simulink model "EDLSim_proj"  (R2022b)
settings: Solver=ode23s  StartTime=0.0  StopTime=tSim  FixedStep=0.01  MaxStep=1e3  RelTol=1e-3  EnableMultiTasking=on
values from neighbouring files (symbols this model uses):
  A = [0 0 v0 ... (first row only)    [main.m]
  Aref = A-B*K    [main.m]
  B = [0;0;1]    [main.m]
  Bref = [0;0;1]    [main.m]
  D = 0.5*rho*Cd*S*v^2    [command.m]    (also in command3.m)
  e0 = 350    [main.m]
  Gama = 1    [main.m]
  Gamar = 1    [main.m]
  Gamat = 1*eye(3)    [main.m]
  Gamax = 1*eye(3)    [main.m]
  gamma0 = deg2rad(-6.6198381)    [main.m]    (also in scaling.m = gamma0/angbar)
  meanDist = 50000    [main.m]
  P = lyap(Aref',Qref)    [main.m]
  phi0 = deg2rad(23.51457)    [main.m]
  psi0 = deg2rad(18.0683)    [main.m]
  r0 = r0*1000    (= 6498270)    [main.m]    (also in scaling.m = 1.0188351238)
  r_des = 10 * 1000    (= 10000)    [main.m]
  r_e = r_e*1000    (= 6378137)    [command.m]    (also in command3.m; main.m; scaling.m = 6378.137)
  Theta = [0 0 1]    [main.m]
  theta0 = deg2rad(174.24384)    [main.m]
  Ts = 0.01    [main.m]
  tSim = T(end)    [main.m]
  v0 = v0*1000    (= 11067.15)    [main.m]    (also in scaling.m = 1)
  varDist = 5000    [main.m]
  x0 = [r0;v0;gamma0]    [main.m]    (also in scaling.m)
settings Model: Creator=Tri  LastModifiedBy=la561195
settings SolverCC: AlgebraicLoopSolver=TrustRegion
settings DataIOCC: LimitDataPoints=on  SaveFormat=Array  ReturnWorkspaceOutputs=off
settings OptimizationCC: LifeSpan=inf
settings DebuggingCC: UnconnectedInputMsg=warning  UnconnectedOutputMsg=warning  UnconnectedLineMsg=warning  SFUnexpectedBacktrackingDiag=warning  SFNoUnconditionalDefaultTransitionDiag=warning  SFExecutionAtInitializationDiag=none  SFMachineParentedDataDiag=warning  ArithmeticOperatorsInVariantConditions=warning
settings HardwareCC: ProdBitPerPointer=32  ProdBitPerSizeT=32  ProdBitPerPtrDiffT=32  ProdLargestAtomicFloat=None  ProdIntDivRoundTo=Undefined  ProdEndianess=Unspecified  ProdWordSize=32  ProdHWDeviceType=32-bit Generic
settings ModelReferenceCC: PropagateSignalLabelsOutOfModel=off
settings SFSimCC: SimUseLocalCustomCode=off  CustomCodeUndefinedFunction=UseInterfaceOnly
settings RTWCC: RTWUseLocalCustomCode=off
settings CodeAppCC: StateflowObjectComments=on
settings GRTTargetCC: TargetLangStandard=C89/C90 (ANSI)
settings ConfigComp: CovMetricSettings=dw  CovSaveCumulativeToWorkspaceVar=on  CovSaveSingleToWorkspaceVar=on  CovExternalEMLEnable=off

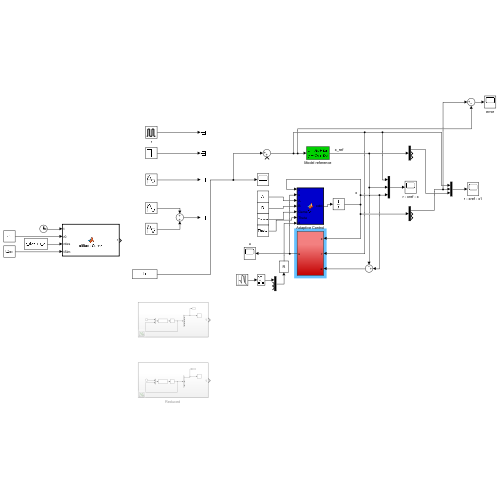
[thumbnail: Simulink's stored preview of the top-level diagram]
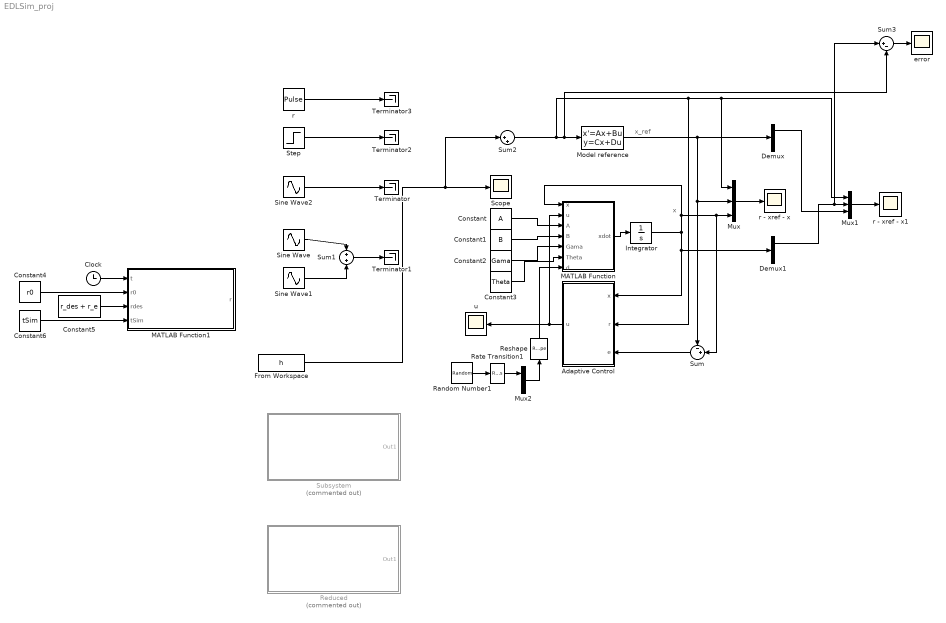
== system EDLSim_proj ==
  note: x
  note: x_ref
  Adaptive Control : Subsystem
  Clock : Clock
  Constant : Constant  Value=A
  Constant1 : Constant  Value=B
  Constant2 : Constant  Value=Gama
  Constant3 : Constant  Value=Theta
  Constant4 : Constant  Value=r0
  Constant5 : Constant  Value=r_des + r_e
  Constant6 : Constant  Value=tSim
  Demux : Demux  Outputs=3
  Demux1 : Demux  Outputs=3
  From Workspace : FromWorkspace  VariableName=h  SampleTime=Ts
  Integrator : Integrator  InitialCondition=x0
  MATLAB Function : MATLAB Function  TreatAsAtomicUnit=on
  MATLAB Function1 : MATLAB Function  TreatAsAtomicUnit=on
  Model reference : StateSpace  A=Aref  B=Bref  C=eye(3)  D=zeros(3,1)  InitialCondition="x0 +  x0 * 0.0001"
  Mux : Mux  Inputs=3
  Mux1 : Mux  Inputs=3
  Mux2 : Mux  Inputs=3
  Random Number1 : RandomNumber  Mean=meanDist  Variance=varDist  Seed=43453  SampleTime=Ts
  Rate Transition1 : RateTransition
  "Reduced " : Subsystem  Commented=on
  Reshape : Reshape  OutputDimensionality=Customize  OutputDimensions=[3,1]
  Scope : Scope
  Sine Wave : Sin  Amplitude=2  Frequency=2*pi/6.25  SampleTime=0
  Sine Wave1 : Sin  Amplitude=3  Frequency=2*pi/10  SampleTime=0
  Sine Wave2 : Sin  Amplitude=r0/84  Bias=r0  Frequency=pi/tSim  Phase=pi/2  SampleTime=0
  Step : Step  Time=5  Before=r0  After=r_e + r_des  SampleTime=0
  Subsystem : Subsystem  Commented=on
  Sum : Sum  Inputs=-+|
  Sum1 : Sum
  Sum2 : Sum  Inputs=|++
  Sum3 : Sum  Inputs=|+-
  Terminator{,1..3} (4 alike) : Terminator
  error : Scope
  r : DiscretePulseGenerator  PulseType=Time based  Amplitude=deg2rad(5)  Period=20  PulseWidth=50
  r - xref - x : Scope
  r - xref - x1 : Scope
  u : Scope
  wires:
  MATLAB Function/1(xdot) -> Integrator/1
  Integrator/1 -> Sum/2, Mux/3, MATLAB Function/1(x), Demux1/1, Adaptive Control/1(x)
  Model reference/1 -> Sum/1, Mux/2, Demux/1
  Mux/1 -> r - xref - x/1
  Sum/1 -> Adaptive Control/3(e)
  Sum1/1 -> Terminator1/1
  Sine Wave2/1 -> Terminator/1
  Sine Wave1/1 -> Sum1/2
  Sine Wave/1 -> Sum1/1
  Step/1 -> Terminator2/1
  Constant1/1 -> MATLAB Function/4(B)
  Constant/1 -> MATLAB Function/3(A)
  Constant2/1 -> MATLAB Function/5(Gama)
  Constant3/1 -> MATLAB Function/6(Theta)
  Sum2/1 -> Model reference/1, Sum3/2, Adaptive Control/2(r), Mux/1, Mux1/1
  r/1 -> Terminator3/1
  Mux1/1 -> r - xref - x1/1
  Adaptive Control/1(u) -> MATLAB Function/2(u), u/1
  Demux1/1 -> Sum3/1, Mux1/2
  Demux/1 -> Mux1/3
  Clock/1 -> MATLAB Function1/1(t)
  Constant4/1 -> MATLAB Function1/2(r0)
  Constant6/1 -> MATLAB Function1/4(tSim)
  Constant5/1 -> MATLAB Function1/3(rdes)
  From Workspace/1 -> Scope/1, Sum2/1
  Random Number1/1 -> Rate Transition1/1
  Mux2/1 -> Reshape/1
  Sum3/1 -> error/1
  Rate Transition1/1 -> Mux2/1
  Reshape/1 -> MATLAB Function/7(d)

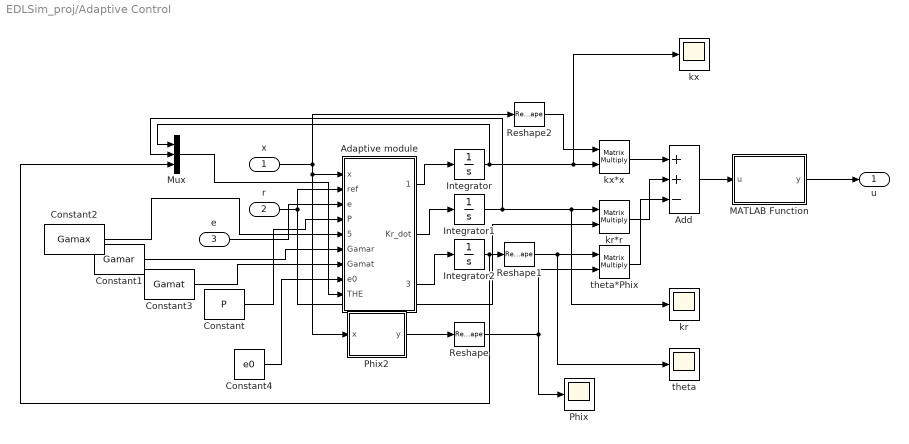
== system EDLSim_proj/Adaptive Control ==
  x : Inport
  r : Inport  Port=2
  e : Inport  Port=3
  Adaptive module : MATLAB Function  TreatAsAtomicUnit=on
  Add : Sum  Inputs=++-
  Constant : Constant  Value=P
  Constant1 : Constant  Value=Gamar
  Constant2 : Constant  Value=Gamax
  Constant3 : Constant  Value=Gamat
  Constant4 : Constant  Value=e0
  Integrator : Integrator
  Integrator1 : Integrator
  Integrator2 : Integrator
  MATLAB Function : MATLAB Function  TreatAsAtomicUnit=on
  Mux : Mux  Inputs=3
  Phix : Scope
  Phix2 : MATLAB Function  TreatAsAtomicUnit=on
  Reshape : Reshape  OutputDimensionality=Column vector (2-D)
  Reshape1 : Reshape  OutputDimensionality=Row vector (2-D)
  Reshape2 : Reshape  OutputDimensionality=Row vector (2-D)
  kr : Scope
  kr*r : Product  Multiplication=Matrix(*)
  kx : Scope
  kx*x : Product  Multiplication=Matrix(*)
  theta : Scope
  theta*Phix : Product  Multiplication=Matrix(*)
  u : Outport
  wires:
  Adaptive module/1(Kx_dot) -> Integrator/1
  kx*x/1 -> Add/1
  kr*r/1 -> Add/2
  theta*Phix/1 -> Add/3
  Integrator2/1 -> Mux/3, Reshape1/1
  Adaptive module/3(Theta_dot) -> Integrator2/1
  Adaptive module/2(Kr_dot) -> Integrator1/1
  Integrator1/1 -> Mux/2, kr/1, kr*r/1
  e/1 -> Adaptive module/3(e)
  x/1 -> Phix2/1(x), Adaptive module/1(x), Reshape2/1
  r/1 -> Adaptive module/2(ref), kr*r/2
  Phix2/1(y) -> Reshape/1
  Reshape/1 -> theta*Phix/2, Phix/1
  Reshape1/1 -> theta/1, theta*Phix/1
  Reshape2/1 -> kx*x/1
  Integrator/1 -> kx/1, kx*x/2, Mux/1
  Constant/1 -> Adaptive module/4(P)
  Constant1/1 -> Adaptive module/6(Gamar)
  Constant2/1 -> Adaptive module/5(Gamax)
  Constant3/1 -> Adaptive module/7(Gamat)
  Add/1 -> MATLAB Function/1(u)
  MATLAB Function/1(y) -> u/1
  Constant4/1 -> Adaptive module/8(e0)
  Mux/1 -> Adaptive module/9(THE)

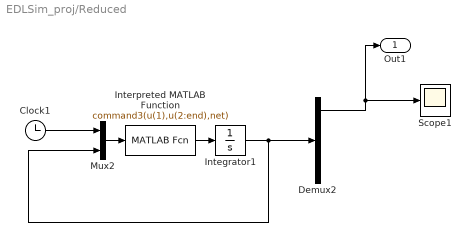
== system EDLSim_proj/Reduced  ==
  Clock1 : Clock
  Demux2 : Demux  Outputs=3
  Integrator1 : Integrator  InitialCondition=[r0;v0;gamma0]
  Interpreted MATLAB Function : MATLABFcn  MATLABFcn=command3(u(1),u(2:end),net)  Output1D=off
  Mux2 : Mux  Inputs=2
  Scope1 : Scope
  Out1 : Outport
  wires:
  Clock1/1 -> Mux2/1
  Interpreted MATLAB Function/1 -> Integrator1/1
  Demux2/1 -> Out1/1, Scope1/1
  Integrator1/1 -> Demux2/1, Mux2/2
  Mux2/1 -> Interpreted MATLAB Function/1

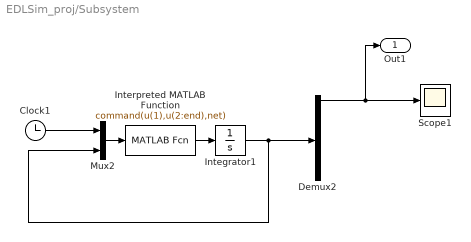
== system EDLSim_proj/Subsystem ==
  Clock1 : Clock
  Demux2 : Demux  Outputs=6
  Integrator1 : Integrator  InitialCondition=[r0;theta0;phi0;v0;gamma0;psi0]
  Interpreted MATLAB Function : MATLABFcn  MATLABFcn=command(u(1),u(2:end),net)
  Mux2 : Mux  Inputs=2
  Scope1 : Scope
  Out1 : Outport
  wires:
  Clock1/1 -> Mux2/1
  Interpreted MATLAB Function/1 -> Integrator1/1
  Demux2/1 -> Out1/1, Scope1/1
  Integrator1/1 -> Demux2/1, Mux2/2
  Mux2/1 -> Interpreted MATLAB Function/1

== matlab function EDLSim_proj/Adaptive Control/Adaptive module ==
  data: x input; Kx_dot output; ref input; Kr_dot output; Theta_dot output; e input; P input; Gamax input; Gamar input; Gamat input; e0 input; THE input
function [Kx_dot,Kr_dot,Theta_dot] = fcn(x,ref,e,P,Gamax,Gamar,Gamat,e0,THE)
% Adaptive parameters
B = [0;0;1];

r = x(1);
v = x(2);
gamma = x(3);

g = 9.81;

Phix = [0;0;-g/v * cos(gamma) + v/r * cos(gamma)];

THE_max = 1e5;

PHIbar = [x; ref; Phix];
%GAMA = [Gamax; Gamar; Gamat];
y = -PHIbar*e'*P*B;

% Projection operator
epsilon = 1;
%THE = [Kx; Kr; Theta];
Proj = zeros(7,1); %%%%%
for ii = 1:length(THE)
        f_THE = (THE(ii)*THE(ii) - THE_max^2)/epsilon/THE_max^2;
        Df_THE = 2*THE(ii)/epsilon/THE_max^2;  
        if f_THE < 0
            Proj(ii) = y(ii);
        elseif (f_THE>=0) && (Df_THE'*y(ii)<=0)
            Proj(ii) = y(ii); 
        elseif (f_THE>=0) && (Df_THE'*y(ii)>0)
            Proj(ii) = y(ii) - Df_THE/norm(Df_THE)*dot((Df_THE'/norm(Df_THE)),y(ii))*f_THE;
        end    
end

% Adaptive laws
if norm(e) > e0
    Kx_dot = Gamax*Proj(1:3); %%%%%%
    Kr_dot = Gamar*Proj(4); %%%%%%
    Theta_dot = Gamat*Proj(5:end); %%%%%%
else 
    Kx_dot   = zeros(3,1);
    Kr_dot   = 0;
    Theta_dot = zeros(3,1);
end

== matlab function EDLSim_proj/MATLAB Function ==
  data: x input; xdot output; u input; A input; B input; Gama input; Theta input; d input
function xdot = fcn(x,u,A,B,Gama,Theta,d)
% System parameters
r = x(1);
v = x(2);
gamma = x(3);

g = 9.81;

Phix = [0;0;-g/v * cos(gamma) + v/r * cos(gamma)];
% Roll dynamics
xdot = A*x + B*Gama*(u+Theta'*Phix) + d;

== matlab function EDLSim_proj/Adaptive Control/Phix2 ==
  data: x input; y output
function y = fcn(x)
%#codegen
r = x(1);
v = x(2);
gamma = x(3);
g = 9.81;
y = [0;0;-g/v * cos(gamma) + v/r * cos(gamma)];

== matlab function EDLSim_proj/MATLAB Function1 ==
  data: t input; r output; r0 input; rdes input; tSim input
function r = altitudeCurve(t, r0, rdes, tSim)
% t: vector of current times
% r0: initial value of r
% rdes: desired value of r
% tSim: total simulation time


% Calculate the time interval for the different stages of the function
tHold = tSim * 2/10; % Time interval for holding r constant at r0
tDecrease = tSim * 6/10; % Time interval for smoothly decreasing r from r0 to rdes

% Calculate the current value of r based on the time elapsed
if t <= tHold % Hold r constant at r0
    r = r0;
elseif t <= (tHold + tDecrease) % Smoothly decrease r from r0 to rdes
    alpha = (t - tHold) / tDecrease; % Calculate the progress of the decrease
    r = (1 - alpha) * r0 + alpha * rdes; % Linearly interpolate r between r0 and rdes
else % Hold r constant at rdes
    r = rdes;
end

end

== matlab function EDLSim_proj/Adaptive Control/MATLAB Function ==
  data: u input; y output
function y = fcn(u)
y = u;
% y = mod(u, 2*pi);
y = 10 * wrapToPi(u);
